simulink model "Quarter_LQRGENA_wh2"  (R2023a)
settings: Solver=ode4  StartTime=0.0  StopTime=10.0  FixedStep=0.002  RelTol=1e-3
values from neighbouring files (symbols this model uses):
  A = [0, 1, 0, -1 ... (first row only)    [GENA_LQR2.m]
  B = [0; 1/ms; 0; -1/mus]    [GENA_LQR2.m]
  B1 = [0;0;-1;cus/mus]    [GENA_LQR2.m]
  C = [1 0 0 0 ... (first row only)    [GENA_LQR2.m]
  D = [0; 1/ms]    [GENA_LQR2.m]
  K = lqr(A,B,Q, R, N)    [GENA_LQR2.m]
libraries: simulink x1
settings Model: Creator=Administrator  LastModifiedBy=Rayna
settings DataIOCC: ReturnWorkspaceOutputs=off
settings DebuggingCC: UnconnectedInputMsg=warning  UnconnectedOutputMsg=warning  UnconnectedLineMsg=warning
settings ModelReferenceCC: EnableRefExpFcnMdlSchedulingChecks=on

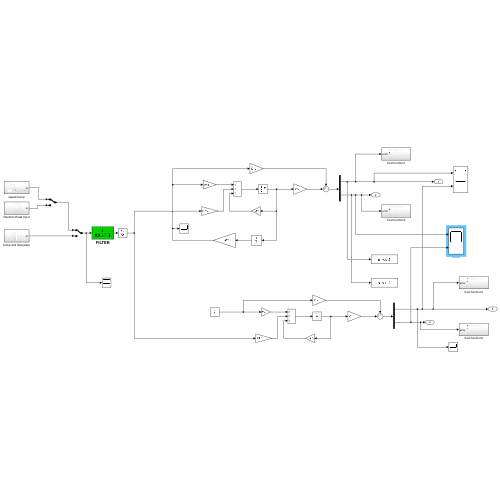
[thumbnail: Simulink's stored preview of the top-level diagram]
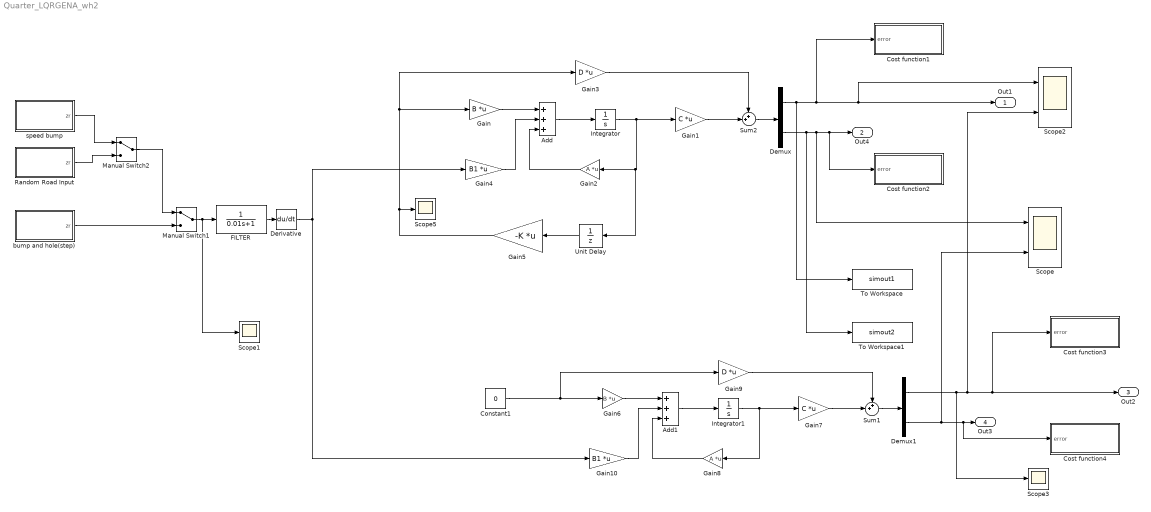
== system Quarter_LQRGENA_wh2 ==
  Add : Sum  Inputs=+++
  Add1 : Sum  Inputs=+++
  Constant1 : Constant  Value=0
  Cost function1 : Subsystem
  Cost function2 : Subsystem
  Cost function3 : Subsystem
  Cost function4 : Subsystem
  Demux : Demux  Outputs=2
  Demux1 : Demux  Outputs=2
  Derivative : Derivative
  FILTER : TransferFcn  Denominator=[0.01 1]
  Gain : Gain  Gain=B  Multiplication=Matrix(K*u)
  Gain1 : Gain  Gain=C  Multiplication=Matrix(K*u)
  Gain10 : Gain  Gain=B1  Multiplication=Matrix(K*u)
  Gain2 : Gain  Gain=A  Multiplication=Matrix(K*u)
  Gain3 : Gain  Gain=D  Multiplication=Matrix(K*u)
  Gain4 : Gain  Gain=B1  Multiplication=Matrix(K*u)
  Gain5 : Gain  Gain=-K  Multiplication=Matrix(K*u)
  Gain6 : Gain  Gain=B  Multiplication=Matrix(K*u)
  Gain7 : Gain  Gain=C  Multiplication=Matrix(K*u)
  Gain8 : Gain  Gain=A  Multiplication=Matrix(K*u)
  Gain9 : Gain  Gain=D  Multiplication=Matrix(K*u)
  Integrator : Integrator  LimitOutput=on  UpperSaturationLimit=10e6  LowerSaturationLimit=-10e6
  Integrator1 : Integrator  UpperSaturationLimit=10e6  LowerSaturationLimit=-10e6
  Manual Switch1 : ManualSwitch
  Manual Switch2 : ManualSwitch
  Random Road Input : Subsystem
  Scope : Scope  NumInputPorts=2
  Scope1 : Scope
  Scope2 : Scope  NumInputPorts=2
  Scope3 : Scope
  Scope5 : Scope
  Sum1 : Sum  Inputs=++|
  Sum2 : Sum  Inputs=++|
  To Workspace : ToWorkspace  VariableName=simout1  SaveFormat=Timeseries  SampleTime=-1
  To Workspace1 : ToWorkspace  VariableName=simout2  SaveFormat=Timeseries  SampleTime=-1
  Unit Delay : UnitDelay  SampleTime=0.002  HasFrameUpgradeWarning=on
  bump and hole(step) : Subsystem
  speed bump : Subsystem
  Out1 : Outport
  Out4 : Outport  Port=2
  Out2 : Outport  Port=3
  Out3 : Outport  Port=4
  wires:
  Gain3/1 -> Sum2/1
  Sum2/1 -> Demux/1
  Gain1/1 -> Sum2/2
  Gain2/1 -> Add/3
  Gain4/1 -> Add/2
  Add/1 -> Integrator/1
  Gain/1 -> Add/1
  Manual Switch1/1 -> Scope1/1, FILTER/1
  Unit Delay/1 -> Gain5/1
  Manual Switch2/1 -> Manual Switch1/1
  FILTER/1 -> Derivative/1
  Integrator/1 -> Unit Delay/1, Gain2/1, Gain1/1
  speed bump/1(zr) -> Manual Switch2/1
  Random Road Input/1(zr) -> Manual Switch2/2
  bump and hole(step)/1(zr) -> Manual Switch1/2
  Gain5/1 -> Scope5/1, Gain/1, Gain3/1
  Gain6/1 -> Add1/1
  Constant1/1 -> Gain9/1, Gain6/1
  Integrator1/1 -> Gain7/1, Gain8/1
  Gain7/1 -> Sum1/2
  Add1/1 -> Integrator1/1
  Derivative/1 -> Gain4/1, Gain10/1
  Gain9/1 -> Sum1/1
  Sum1/1 -> Demux1/1
  Gain10/1 -> Add1/2
  Gain8/1 -> Add1/3
  Demux/1 -> To Workspace/1, Cost function1/1(error), Out1/1, Scope2/1
  Demux/2 -> To Workspace1/1, Scope/1, Cost function2/1(error), Out4/1
  Demux1/2 -> Scope/2, Cost function4/1(error), Out3/1
  Demux1/1 -> Scope3/1, Cost function3/1(error), Out2/1, Scope2/2

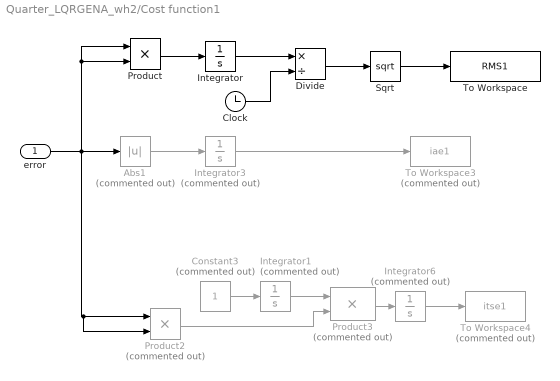
== system Quarter_LQRGENA_wh2/Cost function1 ==
  error : Inport
  Abs1 : Abs  Commented=on
  Clock : Clock
  Constant3 : Constant  Commented=on
  Divide : Product  Inputs=*/
  Integrator : Integrator
  Integrator1 : Integrator  Commented=on
  Integrator3 : Integrator  Commented=on
  Integrator6 : Integrator  Commented=on
  Product : Product
  Product2 : Product  Commented=on
  Product3 : Product  Commented=on  SaturateOnIntegerOverflow=on  OutDataTypeStr=Inherit: Same as first input
  Sqrt : Sqrt
  To Workspace : ToWorkspace  VariableName=RMS1  SampleTime=-1
      settings: MaxDataPoints=1
  To Workspace3 : ToWorkspace  Commented=on  VariableName=iae1  SampleTime=-1
      settings: MaxDataPoints=1
  To Workspace4 : ToWorkspace  Commented=on  VariableName=itse1  SampleTime=-1
      settings: MaxDataPoints=1
  wires:
  Integrator3/1 -> To Workspace3/1
  error/1 -> Product/2, Product/1, Product2/2, Product2/1, Abs1/1
  Abs1/1 -> Integrator3/1
  Integrator1/1 -> Product3/1
  Constant3/1 -> Integrator1/1
  Product2/1 -> Product3/2
  Integrator6/1 -> To Workspace4/1
  Product3/1 -> Integrator6/1
  Product/1 -> Integrator/1
  Integrator/1 -> Divide/1
  Clock/1 -> Divide/2
  Divide/1 -> Sqrt/1
  Sqrt/1 -> To Workspace/1

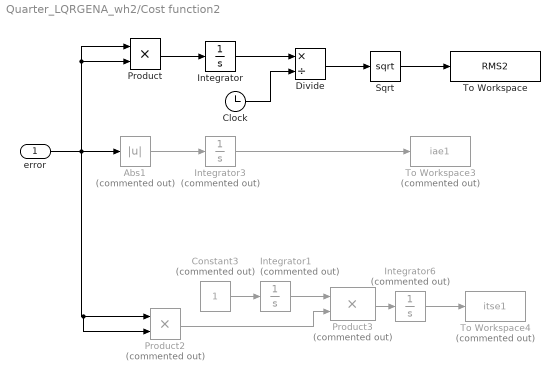
== system Quarter_LQRGENA_wh2/Cost function2 ==
  error : Inport
  Abs1 : Abs  Commented=on
  Clock : Clock
  Constant3 : Constant  Commented=on
  Divide : Product  Inputs=*/
  Integrator : Integrator
  Integrator1 : Integrator  Commented=on
  Integrator3 : Integrator  Commented=on
  Integrator6 : Integrator  Commented=on
  Product : Product
  Product2 : Product  Commented=on
  Product3 : Product  Commented=on  SaturateOnIntegerOverflow=on  OutDataTypeStr=Inherit: Same as first input
  Sqrt : Sqrt
  To Workspace : ToWorkspace  VariableName=RMS2  SampleTime=-1
      settings: MaxDataPoints=1
  To Workspace3 : ToWorkspace  Commented=on  VariableName=iae1  SampleTime=-1
      settings: MaxDataPoints=1
  To Workspace4 : ToWorkspace  Commented=on  VariableName=itse1  SampleTime=-1
      settings: MaxDataPoints=1
  wires:
  Integrator3/1 -> To Workspace3/1
  error/1 -> Product/2, Product/1, Product2/2, Product2/1, Abs1/1
  Abs1/1 -> Integrator3/1
  Integrator1/1 -> Product3/1
  Constant3/1 -> Integrator1/1
  Product2/1 -> Product3/2
  Integrator6/1 -> To Workspace4/1
  Product3/1 -> Integrator6/1
  Product/1 -> Integrator/1
  Integrator/1 -> Divide/1
  Clock/1 -> Divide/2
  Divide/1 -> Sqrt/1
  Sqrt/1 -> To Workspace/1

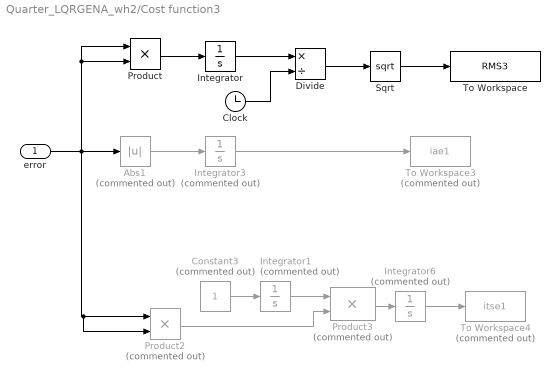
== system Quarter_LQRGENA_wh2/Cost function3 ==
  error : Inport
  Abs1 : Abs  Commented=on
  Clock : Clock
  Constant3 : Constant  Commented=on
  Divide : Product  Inputs=*/
  Integrator : Integrator
  Integrator1 : Integrator  Commented=on
  Integrator3 : Integrator  Commented=on
  Integrator6 : Integrator  Commented=on
  Product : Product
  Product2 : Product  Commented=on
  Product3 : Product  Commented=on  SaturateOnIntegerOverflow=on  OutDataTypeStr=Inherit: Same as first input
  Sqrt : Sqrt
  To Workspace : ToWorkspace  VariableName=RMS3  SampleTime=-1
      settings: MaxDataPoints=1
  To Workspace3 : ToWorkspace  Commented=on  VariableName=iae1  SampleTime=-1
      settings: MaxDataPoints=1
  To Workspace4 : ToWorkspace  Commented=on  VariableName=itse1  SampleTime=-1
      settings: MaxDataPoints=1
  wires:
  Integrator3/1 -> To Workspace3/1
  error/1 -> Product/2, Product/1, Product2/2, Product2/1, Abs1/1
  Abs1/1 -> Integrator3/1
  Integrator1/1 -> Product3/1
  Constant3/1 -> Integrator1/1
  Product2/1 -> Product3/2
  Integrator6/1 -> To Workspace4/1
  Product3/1 -> Integrator6/1
  Product/1 -> Integrator/1
  Integrator/1 -> Divide/1
  Clock/1 -> Divide/2
  Divide/1 -> Sqrt/1
  Sqrt/1 -> To Workspace/1

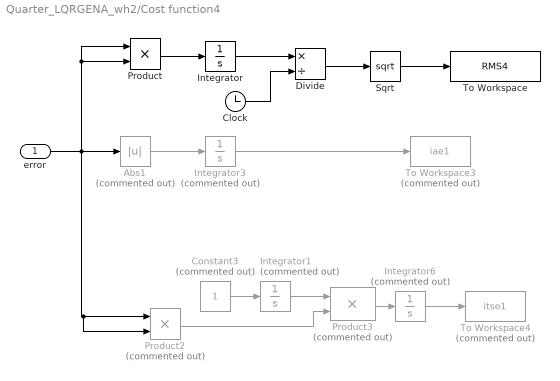
== system Quarter_LQRGENA_wh2/Cost function4 ==
  error : Inport
  Abs1 : Abs  Commented=on
  Clock : Clock
  Constant3 : Constant  Commented=on
  Divide : Product  Inputs=*/
  Integrator : Integrator
  Integrator1 : Integrator  Commented=on
  Integrator3 : Integrator  Commented=on
  Integrator6 : Integrator  Commented=on
  Product : Product
  Product2 : Product  Commented=on
  Product3 : Product  Commented=on  SaturateOnIntegerOverflow=on  OutDataTypeStr=Inherit: Same as first input
  Sqrt : Sqrt
  To Workspace : ToWorkspace  VariableName=RMS4  SampleTime=-1
      settings: MaxDataPoints=1
  To Workspace3 : ToWorkspace  Commented=on  VariableName=iae1  SampleTime=-1
      settings: MaxDataPoints=1
  To Workspace4 : ToWorkspace  Commented=on  VariableName=itse1  SampleTime=-1
      settings: MaxDataPoints=1
  wires:
  Integrator3/1 -> To Workspace3/1
  error/1 -> Product/2, Product/1, Product2/2, Product2/1, Abs1/1
  Abs1/1 -> Integrator3/1
  Integrator1/1 -> Product3/1
  Constant3/1 -> Integrator1/1
  Product2/1 -> Product3/2
  Integrator6/1 -> To Workspace4/1
  Product3/1 -> Integrator6/1
  Product/1 -> Integrator/1
  Integrator/1 -> Divide/1
  Clock/1 -> Divide/2
  Divide/1 -> Sqrt/1
  Sqrt/1 -> To Workspace/1

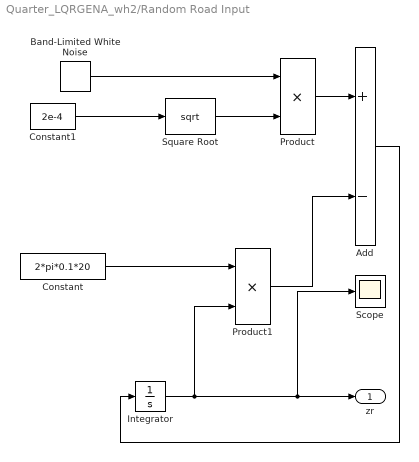
== system Quarter_LQRGENA_wh2/Random Road Input ==
  Add : Sum  Inputs=+-
  Band-Limited White Noise : simulink/Sources/Band-Limited White Noise  Cov=[0.1]  Ts=0.002  seed=[23341]
  Constant : Constant  Value=2*pi*0.1*20
  Constant1 : Constant  Value=2e-4
  Integrator : Integrator
  Product : Product
  Product1 : Product
  Scope : Scope
  Square Root : Sqrt
  zr : Outport
  wires:
  Band-Limited White Noise/1 -> Product/1
  Product/1 -> Add/1
  Product1/1 -> Add/2
  Integrator/1 -> Scope/1, zr/1, Product1/2
  Add/1 -> Integrator/1
  Constant/1 -> Product1/1
  Square Root/1 -> Product/2
  Constant1/1 -> Square Root/1

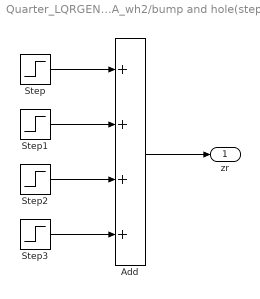
== system Quarter_LQRGENA_wh2/bump and hole(step) ==
  Add : Sum  Inputs=++++
  Step : Step  After=0.05  SampleTime=0
  Step1 : Step  Time=2  After=-0.05  SampleTime=0
  Step2 : Step  Time=5  After=-0.05  SampleTime=0
  Step3 : Step  Time=6  After=0.05  SampleTime=0
  zr : Outport
  wires:
  Step3/1 -> Add/4
  Step2/1 -> Add/3
  Step/1 -> Add/1
  Step1/1 -> Add/2
  Add/1 -> zr/1

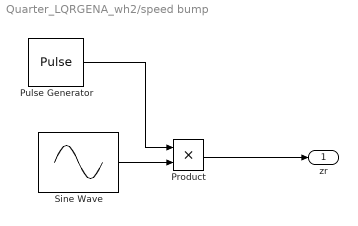
== system Quarter_LQRGENA_wh2/speed bump ==
  Product : Product
  Pulse Generator : DiscretePulseGenerator  PulseType=Time based  Period=3  PulseWidth=10/3  PhaseDelay=2
  Sine Wave : Sin  Amplitude=0.08  Frequency=10*pi
  zr : Outport
  wires:
  Sine Wave/1 -> Product/2
  Pulse Generator/1 -> Product/1
  Product/1 -> zr/1
